simulink model "FailureAnalysis"  (R2018b)
settings: Solver=VariableStepAuto  StartTime=0.0  StopTime=10.0  RelTol=1e-3
libraries: powerlib x75, peGeneralControl x6, dspstat3 x6, sldrtlib x1
settings Model: Creator=hp  LastModifiedBy=hp

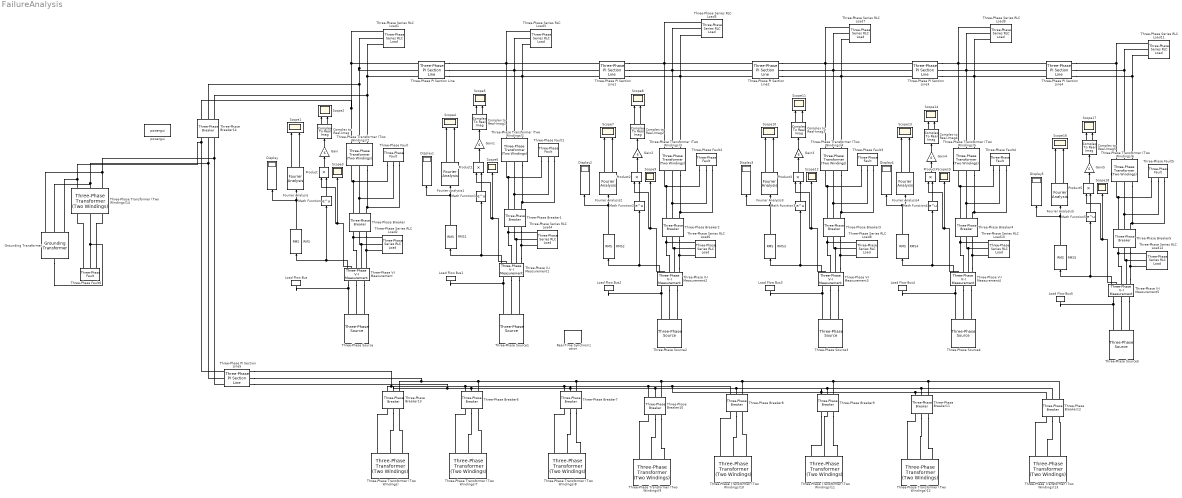
== system FailureAnalysis ==
  Complex to Real-Imag{,1..5} (6 alike) : ComplexToRealImag
  Display{,1..5} (6 alike) : Display
  Fourier Analysis{,1..5} (6 alike) : peGeneralControl/Fourier Analysis  f=60  n=[1 2]  M0=1  Ph0=0  Ts=-1
  Gain{,1..5} (6 alike) : Gain  Gain=6
  "Grounding Transformer " : powerlib/Elements/Grounding Transformer   UNITS=pu  NominalPower="[100e6   60]"  NominalVoltage=25e3  ZeroSequenceImpedance_pu=[0.025 0.75]  MagnetizationBranch_pu=[500 500]  ZeroSequenceImpedance_SI=[0.052083 589.05]  MagnetizationBranch_SI=[1041.7 3.927e+005]  Measurements=None
      settings: SourceProductName=Simscape Power Systems  SourceProductBaseCode=PS
  Load Flow Bus : powerlib/Measurements/Load Flow Bus  LConnTagsString=a  Phases=single  Connectors=on one side  ID=BUS_1  Vbase=25e3  Vref=1  Vangle=0  VLF=1  VLFb=1  VLFc=1  angleLF=0  angleLFb=0  angleLFc=0
      settings: SourceProductName=Simscape Power Systems
  Load Flow Bus1 : powerlib/Measurements/Load Flow Bus  LConnTagsString=a  Phases=single  Connectors=on one side  ID=BUS_2  Vbase=25e3  Vref=1  Vangle=0  VLF=1  VLFb=1  VLFc=1  angleLF=0  angleLFb=0  angleLFc=0
      settings: SourceProductName=Simscape Power Systems
  Load Flow Bus2 : powerlib/Measurements/Load Flow Bus  LConnTagsString=a  Phases=single  Connectors=on one side  ID=BUS_3  Vbase=25e3  Vref=1  Vangle=0  VLF=1  VLFb=1  VLFc=1  angleLF=0  angleLFb=0  angleLFc=0
      settings: SourceProductName=Simscape Power Systems
  Load Flow Bus3 : powerlib/Measurements/Load Flow Bus  LConnTagsString=a  Phases=single  Connectors=on one side  ID=BUS_4  Vbase=25e3  Vref=1  Vangle=0  VLF=1  VLFb=1  VLFc=1  angleLF=0  angleLFb=0  angleLFc=0
      settings: SourceProductName=Simscape Power Systems
  Load Flow Bus4 : powerlib/Measurements/Load Flow Bus  LConnTagsString=a  Phases=single  Connectors=on one side  ID=BUS_5  Vbase=25e3  Vref=1  Vangle=0  VLF=1  VLFb=1  VLFc=1  angleLF=0  angleLFb=0  angleLFc=0
      settings: SourceProductName=Simscape Power Systems
  Load Flow Bus5 : powerlib/Measurements/Load Flow Bus  LConnTagsString=a  Phases=single  Connectors=on one side  ID=BUS_6  Vbase=25e3  Vref=1  Vangle=0  VLF=1  VLFb=1  VLFc=1  angleLF=0  angleLFb=0  angleLFc=0
      settings: SourceProductName=Simscape Power Systems
  Math Function{,1..5} (6 alike) : Math  SaturateOnIntegerOverflow=on
  Product{,1..5} (6 alike) : Product
  RMS{,1..5} (6 alike) : dspstat3/RMS  run=off  directionMode=Each column  dimension=1  InputProcessing=Columns as channels (frame based)  reset_popup=None
  Real-Time Synchronization : sldrtlib/Real-Time Synchronization  SampleTime=0.1  MaxMissedTicks=10  ShowMissedTicks=off  YieldWhenWaiting=off
  Scope{1..2,4..5,7..8,10..11,13..14,16..17} (12 alike) : Scope  NumInputPorts=2
  Scope{3,6,9,12,15,18} (6 alike) : Scope
  Three-Phase PI Section Line{,1..4} (5 alike) : powerlib/Elements/Three-Phase PI Section Line  LConnTagsString=a|b|c  RConnTagsString=A|B|C  Frequency=60  Resistances=[ 0.01273 0.3864]  Inductances="[ 0.9337e-3  4.1264e-3]"  Capacitances=[12.74e-9 7.751e-9]  Length=0.1
      settings: SourceProductName=Simscape Power Systems
  Three-Phase PI Section Line5 : powerlib/Elements/Three-Phase PI Section Line  LConnTagsString=a|b|c  RConnTagsString=A|B|C  Frequency=60  Resistances=[ 0.01273 0.3864]  Inductances="[ 0.9337e-3  4.1264e-3]"  Capacitances=[12.74e-9 7.751e-9]  Length=100
      settings: SourceProductName=Simscape Power Systems
  Three-Phase Series RLC Load{1..12} (12 alike) : powerlib/Elements/Three-Phase Series RLC Load  LConnTagsString=A|B|C  Configuration=Y (grounded)  NominalVoltage=(1000)*10.749  Vabc=[1e3 1e3 1e3]  Vabcp=[1e3 1e3 1e3]  NominalFrequency=60  UnbalancedPower=off  ActivePower=10e3  InductivePower=100  CapacitivePower=100  Pabc=[10e3 9e3 11e3]  QLabc=[100 90 110]  QCabc=[100 90 110]  Pabcp=[10e3 9e3 11e3]  QLabcp=[100 90 110]  QCabcp=[100 90 110]  Measurements=Branch voltages and currents  LoadType=constant PQ
  Three-Phase Transformer (Two Windings){,7..13} (8 alike) : powerlib/Elements/Three-Phase Transformer (Two Windings)  Winding1Connection=Yg  Winding2Connection=Yg  CoreType=Three single-phase transformers  SetSaturation=off  Hysteresis=off  DataFile='hysteresis'  SetInitialFlux=off  Measurements=None  UNITS=pu  NominalPower=[ 250e6 , 60 ]  Winding1=[ 735e3 , 0.002 , 0.08 ]  Winding2=[ 315e3 , 0.002 , 0.08 ]  Rm=500  Lm=500  L0=0.5  Saturation=[ 0,0 ; 0.0024,1.2 ; 1.0,1.52 ]  InitialFluxes=[ 0.8 , -0.8 , 0.7 ]  MoreParameters=off  BreakLoop=off  DataType=off  TransfoNumber=1
  Three-Phase Transformer (Two Windings){1..6} (6 alike) : powerlib/Elements/Three-Phase Transformer (Two Windings)  Winding1Connection=Yg  Winding2Connection=Yg  CoreType=Three single-phase transformers  SetSaturation=off  Hysteresis=off  DataFile='hysteresis'  SetInitialFlux=off  Measurements=All measurements (V I Fluxes)  UNITS=pu  NominalPower=[ 250e6 , 60 ]  Winding1=[ 735e3 , 0.002 , 0.08 ]  Winding2=[ 315e3 , 0.002 , 0.08 ]  Rm=500  Lm=500  L0=0.5  Saturation=[ 0,0 ; 0.0024,1.2 ; 1.0,1.52 ]  InitialFluxes=[ 0.8 , -0.8 , 0.7 ]  MoreParameters=off  BreakLoop=off  DataType=off  TransfoNumber=1
  Three-Phase Transformer (Two Windings)14 : powerlib/Elements/Three-Phase Transformer (Two Windings)  Winding1Connection=Yg  Winding2Connection=Yg  CoreType=Three single-phase transformers  SetSaturation=off  Hysteresis=off  DataFile='hysteresis'  SetInitialFlux=off  Measurements=None  UNITS=pu  NominalPower=[ 250e6 , 60 ]  Winding1=[ 17.5e3 , 0.002 , 0.08 ]  Winding2=[ 120 , 0.002 , 0.08 ]  Rm=500  Lm=500  L0=0.5  Saturation=[ 0,0 ; 0.0024,1.2 ; 1.0,1.52 ]  InitialFluxes=[ 0.8 , -0.8 , 0.7 ]  MoreParameters=off  BreakLoop=off  DataType=off  TransfoNumber=1
  Three-Phase V-I Measurement{,1..5} (6 alike) : powerlib/Measurements/Three-Phase V-I Measurement  VoltageMeasurement=phase-to-ground  SetLabelV=off  LabelV=Vabc  Vpu=on  VpuLL=off  CurrentMeasurement=yes  SetLabelI=off  LabelI=Iabc  Ipu=off  Pbase=100e6  Vbase=500e3  OutputType=Complex  PhasorSimulation=off  PSBequivalent=0
  Three-Phase Breaker{,1..14} (15 alike) : powerlib/Elements/Three-Phase Breaker  InitialState=closed  SwitchA=on  SwitchB=on  SwitchC=on  SwitchTimes="[1/60  5/60]"  External=off  BreakerResistance=0.01  SnubberResistance=1e6  SnubberCapacitance=inf  Measurements=None
  Three-Phase Fault{,1..5} (6 alike) : powerlib/Elements/Three-Phase Fault  InitialStates=0  FaultA=on  FaultB=on  FaultC=on  GroundFault=on  SwitchTimes="[1/60  5/60]"  External=off  SwitchStatus=NaN  FaultResistance=0.001  GroundResistance=0.01  SnubberResistance=1e6  SnubberCapacitance=inf  Measurements=Fault voltages
  Three-Phase Fault6 : powerlib/Elements/Three-Phase Fault  InitialStates=0  FaultA=on  FaultB=on  FaultC=on  GroundFault=on  SwitchTimes="[1/60  5/60]"  External=off  SwitchStatus=NaN  FaultResistance=0.001  GroundResistance=0.01  SnubberResistance=1e6  SnubberCapacitance=inf  Measurements=None
  Three-Phase Source{,1..5} (6 alike) : powerlib/Electrical Sources/Three-Phase Source  InternalConnection=Yg  VoltagePhases=off  Voltage=(25000)*0.999949  PhaseAngle=0.0058776  Voltage_phases=[25e3 25e3 25e3]/sqrt(3)  PhaseAngles_phases=[0 -120 +120]  Frequency=60  NonIdealSource=on  SpecifyImpedance=off  Resistance=0.8929  Inductance=16.58e-3  ShortCircuitLevel=100e6  BaseVoltage=25e3  XRratio=7  BusType=swing  Pref=7e6  Qref=0  Prefabc=[10e3, 10e3, 10e3]  Qrefabc=[0, 0, 0]  Qmin=-inf  Qmax=inf
  powergui : powerlib/powergui  Priority=1  SimulationMode=Continuous  SampleTime=50e-6  frequency=60  Iterations=50  frequencyindice=60  Pbase=7e6  ErrMax=0.0001  UnitsV=kV  UnitsW=MW  buscounter=0  FunctionMessages=off  echomessages=off  EnableUseOfTLC=off  CurrentSourceSwitches=off  DisableSnubberDevices=off  DisableRonSwitches=off  DisableVfSwitches=off  DisplayEquations=off  SolverType=Tustin/Backward Euler (TBE)  Interpol=off  ExternalGateDelay=off  methode=off  Ts=100  x0status=blocks  SPID=on  SwTol=0  HookPort=off  RestoreLinks=warning  ResistiveCurrentMeasurement=off  Frange=[0:2:500]  Ylog=off  Xlog=on  ShowGrid=off  save=off  variable=ZData  structure=0  ZoomFFT=off  StartTime=0.0  cycles=1  DisplayStyle=1  fundamental=60  FreqAxis=off  MaxFrequency=1000  frequencyindicesteady=60  RmsSteady=1  display=off
  wires:
  Math Function/1 -> Product/2
  Gain/1 -> Complex to Real-Imag/1
  Product/1 -> Gain/1
  RMS/1 -> Display/1, Fourier Analysis/1
  Fourier Analysis/2 -> Scope1/2
  Fourier Analysis/1 -> Scope1/1
  Complex to Real-Imag/1 -> Scope2/1
  Complex to Real-Imag/2 -> Scope2/2
  Three-Phase V-I Measurement/1 -> Math Function/1, RMS/1
  Three-Phase V-I Measurement/2 -> Product/1, Scope3/1
  Gain1/1 -> Complex to Real-Imag1/1
  Three-Phase V-I Measurement1/2 -> Product1/1, Scope6/1
  Three-Phase V-I Measurement1/1 -> Math Function1/1, RMS1/1
  Fourier Analysis1/1 -> Scope4/1
  Product1/1 -> Gain1/1
  Complex to Real-Imag1/1 -> Scope5/1
  Complex to Real-Imag1/2 -> Scope5/2
  Math Function1/1 -> Product1/2
  RMS1/1 -> Display1/1, Fourier Analysis1/1
  Fourier Analysis1/2 -> Scope4/2
  Gain2/1 -> Complex to Real-Imag2/1
  Three-Phase V-I Measurement2/2 -> Product2/1, Scope9/1
  Three-Phase V-I Measurement2/1 -> Math Function2/1, RMS2/1
  Fourier Analysis2/1 -> Scope7/1
  Product2/1 -> Gain2/1
  Complex to Real-Imag2/1 -> Scope8/1
  Complex to Real-Imag2/2 -> Scope8/2
  Math Function2/1 -> Product2/2
  RMS2/1 -> Display2/1, Fourier Analysis2/1
  Fourier Analysis2/2 -> Scope7/2
  Gain3/1 -> Complex to Real-Imag3/1
  Three-Phase V-I Measurement3/2 -> Product3/1, Scope12/1
  Three-Phase V-I Measurement3/1 -> Math Function3/1, RMS3/1
  Fourier Analysis3/1 -> Scope10/1
  Product3/1 -> Gain3/1
  Complex to Real-Imag3/1 -> Scope11/1
  Complex to Real-Imag3/2 -> Scope11/2
  Math Function3/1 -> Product3/2
  RMS3/1 -> Display3/1, Fourier Analysis3/1
  Fourier Analysis3/2 -> Scope10/2
  Math Function4/1 -> Product4/2
  Three-Phase V-I Measurement4/1 -> Math Function4/1, RMS4/1
  Fourier Analysis4/2 -> Scope13/2
  Product4/1 -> Gain4/1
  Complex to Real-Imag4/2 -> Scope14/2
  Three-Phase V-I Measurement4/2 -> Product4/1, Scope15/1
  RMS4/1 -> Display4/1, Fourier Analysis4/1
  Gain4/1 -> Complex to Real-Imag4/1
  Fourier Analysis4/1 -> Scope13/1
  Complex to Real-Imag4/1 -> Scope14/1
  Math Function5/1 -> Product5/2
  Three-Phase V-I Measurement5/1 -> Math Function5/1, RMS5/1
  Fourier Analysis5/2 -> Scope16/2
  Product5/1 -> Gain5/1
  Complex to Real-Imag5/2 -> Scope17/2
  Three-Phase V-I Measurement5/2 -> Product5/1, Scope18/1
  RMS5/1 -> Display5/1, Fourier Analysis5/1
  Gain5/1 -> Complex to Real-Imag5/1
  Fourier Analysis5/1 -> Scope16/1
  Complex to Real-Imag5/1 -> Scope17/1
  connections:
  Three-Phase V-I Measurement/LConn1 -- Three-Phase Source/RConn1 -- Load Flow Bus/LConn1
  Three-Phase V-I Measurement/LConn2 -- Three-Phase Source/RConn2
  Three-Phase V-I Measurement/LConn3 -- Three-Phase Source/RConn3
  Three-Phase Breaker/LConn3 -- Three-Phase Series RLC Load2/LConn3 -- Three-Phase V-I Measurement/RConn3
  Three-Phase V-I Measurement/RConn2 -- Three-Phase Breaker/LConn2 -- Three-Phase Series RLC Load2/LConn2
  Three-Phase Breaker/LConn1 -- Three-Phase V-I Measurement/RConn1 -- Three-Phase Series RLC Load2/LConn1
  Three-Phase Transformer (Two Windings)2/LConn3 -- Three-Phase Breaker/RConn3 -- Three-Phase Fault/LConn3
  Three-Phase Breaker/RConn2 -- Three-Phase Transformer (Two Windings)2/LConn2 -- Three-Phase Fault/LConn2
  Three-Phase Breaker/RConn1 -- Three-Phase Transformer (Two Windings)2/LConn1 -- Three-Phase Fault/LConn1
  Three-Phase Series RLC Load1/LConn2 -- Three-Phase PI Section Line/LConn2 -- Three-Phase Breaker14/RConn2 -- Three-Phase Transformer (Two Windings)2/RConn2
  Three-Phase Transformer (Two Windings)2/RConn1 -- Three-Phase Breaker14/RConn1 -- Three-Phase PI Section Line/LConn1 -- Three-Phase Series RLC Load1/LConn1
  Three-Phase Transformer (Two Windings)2/RConn3 -- Three-Phase Breaker14/RConn3 -- Three-Phase PI Section Line/LConn3 -- Three-Phase Series RLC Load1/LConn3
  Three-Phase Fault1/LConn3 -- Three-Phase Transformer (Two Windings)1/LConn3 -- Three-Phase Breaker1/RConn3
  Three-Phase Fault1/LConn2 -- Three-Phase Breaker1/RConn2 -- Three-Phase Transformer (Two Windings)1/LConn2
  Three-Phase V-I Measurement1/RConn3 -- Three-Phase Breaker1/LConn3 -- Three-Phase Series RLC Load4/LConn3
  Three-Phase Series RLC Load4/LConn2 -- Three-Phase Breaker1/LConn2 -- Three-Phase V-I Measurement1/RConn2
  Three-Phase Fault1/LConn1 -- Three-Phase Transformer (Two Windings)1/LConn1 -- Three-Phase Breaker1/RConn1
  Three-Phase Series RLC Load4/LConn1 -- Three-Phase V-I Measurement1/RConn1 -- Three-Phase Breaker1/LConn1
  Load Flow Bus1/LConn1 -- Three-Phase V-I Measurement1/LConn1 -- Three-Phase Source1/RConn1
  Three-Phase Transformer (Two Windings)1/RConn1 -- Three-Phase PI Section Line1/LConn1 -- Three-Phase Series RLC Load3/LConn1 -- Three-Phase PI Section Line/RConn1
  Three-Phase V-I Measurement1/LConn3 -- Three-Phase Source1/RConn3
  Three-Phase Transformer (Two Windings)1/RConn3 -- Three-Phase PI Section Line1/LConn3 -- Three-Phase PI Section Line/RConn3 -- Three-Phase Series RLC Load3/LConn3
  Three-Phase V-I Measurement1/LConn2 -- Three-Phase Source1/RConn2
  Three-Phase Series RLC Load3/LConn2 -- Three-Phase Transformer (Two Windings)1/RConn2 -- Three-Phase PI Section Line1/LConn2 -- Three-Phase PI Section Line/RConn2
  Three-Phase Fault2/LConn3 -- Three-Phase Transformer (Two Windings)3/LConn3 -- Three-Phase Breaker2/RConn3
  Three-Phase Fault2/LConn2 -- Three-Phase Breaker2/RConn2 -- Three-Phase Transformer (Two Windings)3/LConn2
  Three-Phase V-I Measurement2/RConn3 -- Three-Phase Breaker2/LConn3 -- Three-Phase Series RLC Load6/LConn3
  Three-Phase Series RLC Load6/LConn2 -- Three-Phase Breaker2/LConn2 -- Three-Phase V-I Measurement2/RConn2
  Three-Phase Fault2/LConn1 -- Three-Phase Transformer (Two Windings)3/LConn1 -- Three-Phase Breaker2/RConn1
  Three-Phase Series RLC Load6/LConn1 -- Three-Phase V-I Measurement2/RConn1 -- Three-Phase Breaker2/LConn1
  Load Flow Bus2/LConn1 -- Three-Phase V-I Measurement2/LConn1 -- Three-Phase Source2/RConn1
  Three-Phase Transformer (Two Windings)3/RConn1 -- Three-Phase Series RLC Load5/LConn1 -- Three-Phase PI Section Line2/LConn1 -- Three-Phase PI Section Line1/RConn1
  Three-Phase V-I Measurement2/LConn3 -- Three-Phase Source2/RConn3
  Three-Phase Transformer (Two Windings)3/RConn3 -- Three-Phase PI Section Line2/LConn3 -- Three-Phase PI Section Line1/RConn3 -- Three-Phase Series RLC Load5/LConn3
  Three-Phase V-I Measurement2/LConn2 -- Three-Phase Source2/RConn2
  Three-Phase Series RLC Load5/LConn2 -- Three-Phase Transformer (Two Windings)3/RConn2 -- Three-Phase PI Section Line2/LConn2 -- Three-Phase PI Section Line1/RConn2
  Three-Phase Fault3/LConn3 -- Three-Phase Transformer (Two Windings)4/LConn3 -- Three-Phase Breaker3/RConn3
  Three-Phase Fault3/LConn2 -- Three-Phase Breaker3/RConn2 -- Three-Phase Transformer (Two Windings)4/LConn2
  Three-Phase V-I Measurement3/RConn3 -- Three-Phase Breaker3/LConn3 -- Three-Phase Series RLC Load8/LConn3
  Three-Phase Series RLC Load8/LConn2 -- Three-Phase Breaker3/LConn2 -- Three-Phase V-I Measurement3/RConn2
  Three-Phase Fault3/LConn1 -- Three-Phase Transformer (Two Windings)4/LConn1 -- Three-Phase Breaker3/RConn1
  Three-Phase Series RLC Load8/LConn1 -- Three-Phase V-I Measurement3/RConn1 -- Three-Phase Breaker3/LConn1
  Load Flow Bus3/LConn1 -- Three-Phase V-I Measurement3/LConn1 -- Three-Phase Source3/RConn1
  Three-Phase Transformer (Two Windings)4/RConn1 -- Three-Phase Series RLC Load7/LConn1 -- Three-Phase PI Section Line3/LConn1 -- Three-Phase PI Section Line2/RConn1
  Three-Phase V-I Measurement3/LConn3 -- Three-Phase Source3/RConn3
  Three-Phase Transformer (Two Windings)4/RConn3 -- Three-Phase PI Section Line3/LConn3 -- Three-Phase PI Section Line2/RConn3 -- Three-Phase Series RLC Load7/LConn3
  Three-Phase V-I Measurement3/LConn2 -- Three-Phase Source3/RConn2
  Three-Phase Series RLC Load7/LConn2 -- Three-Phase Transformer (Two Windings)4/RConn2 -- Three-Phase PI Section Line3/LConn2 -- Three-Phase PI Section Line2/RConn2
  Three-Phase V-I Measurement4/RConn3 -- Three-Phase Breaker4/LConn3 -- Three-Phase Series RLC Load10/LConn3
  Three-Phase Series RLC Load10/LConn1 -- Three-Phase Breaker4/LConn1 -- Three-Phase V-I Measurement4/RConn1
  Load Flow Bus4/LConn1 -- Three-Phase V-I Measurement4/LConn1 -- Three-Phase Source4/RConn1
  Three-Phase Fault4/LConn3 -- Three-Phase Transformer (Two Windings)5/LConn3 -- Three-Phase Breaker4/RConn3
  Three-Phase Series RLC Load10/LConn2 -- Three-Phase V-I Measurement4/RConn2 -- Three-Phase Breaker4/LConn2
  Three-Phase Fault4/LConn2 -- Three-Phase Breaker4/RConn2 -- Three-Phase Transformer (Two Windings)5/LConn2
  Three-Phase Fault4/LConn1 -- Three-Phase Breaker4/RConn1 -- Three-Phase Transformer (Two Windings)5/LConn1
  Three-Phase V-I Measurement4/LConn3 -- Three-Phase Source4/RConn3
  Three-Phase Transformer (Two Windings)5/RConn3 -- Three-Phase PI Section Line4/LConn3 -- Three-Phase PI Section Line3/RConn3 -- Three-Phase Series RLC Load9/LConn3
  Three-Phase Series RLC Load9/LConn2 -- Three-Phase Transformer (Two Windings)5/RConn2 -- Three-Phase PI Section Line4/LConn2 -- Three-Phase PI Section Line3/RConn2
  Three-Phase Transformer (Two Windings)5/RConn1 -- Three-Phase PI Section Line4/LConn1 -- Three-Phase PI Section Line3/RConn1 -- Three-Phase Series RLC Load9/LConn1
  Three-Phase V-I Measurement4/LConn2 -- Three-Phase Source4/RConn2
  Three-Phase V-I Measurement5/RConn3 -- Three-Phase Breaker5/LConn3 -- Three-Phase Series RLC Load12/LConn3
  Three-Phase Series RLC Load12/LConn1 -- Three-Phase Breaker5/LConn1 -- Three-Phase V-I Measurement5/RConn1
  Load Flow Bus5/LConn1 -- Three-Phase V-I Measurement5/LConn1 -- Three-Phase Source5/RConn1
  Three-Phase Fault5/LConn3 -- Three-Phase Transformer (Two Windings)6/LConn3 -- Three-Phase Breaker5/RConn3
  Three-Phase Series RLC Load12/LConn2 -- Three-Phase V-I Measurement5/RConn2 -- Three-Phase Breaker5/LConn2
  Three-Phase Fault5/LConn2 -- Three-Phase Breaker5/RConn2 -- Three-Phase Transformer (Two Windings)6/LConn2
  Three-Phase Fault5/LConn1 -- Three-Phase Breaker5/RConn1 -- Three-Phase Transformer (Two Windings)6/LConn1
  Three-Phase V-I Measurement5/LConn3 -- Three-Phase Source5/RConn3
  Three-Phase Transformer (Two Windings)6/RConn3 -- Three-Phase PI Section Line4/RConn3 -- Three-Phase Series RLC Load11/LConn3
  Three-Phase Series RLC Load11/LConn2 -- Three-Phase PI Section Line4/RConn2 -- Three-Phase Transformer (Two Windings)6/RConn2
  Three-Phase Transformer (Two Windings)6/RConn1 -- Three-Phase Series RLC Load11/LConn1 -- Three-Phase PI Section Line4/RConn1
  Three-Phase V-I Measurement5/LConn2 -- Three-Phase Source5/RConn2
  Three-Phase Breaker6/RConn1 -- Three-Phase PI Section Line5/LConn1 -- Three-Phase Breaker13/RConn1 -- Three-Phase Breaker9/RConn1 -- Three-Phase Breaker12/RConn1 -- Three-Phase Breaker11/RConn1 -- Three-Phase Breaker8/RConn1 -- Three-Phase Breaker10/RConn1 -- Three-Phase Breaker7/RConn1
  Three-Phase Breaker7/RConn3 -- Three-Phase PI Section Line5/LConn2 -- Three-Phase Breaker13/RConn3 -- Three-Phase Breaker6/RConn3 -- Three-Phase Breaker12/RConn3 -- Three-Phase Breaker11/RConn3 -- Three-Phase Breaker9/RConn3 -- Three-Phase Breaker8/RConn3 -- Three-Phase Breaker10/RConn3
  Three-Phase Breaker8/RConn2 -- Three-Phase Breaker12/RConn2 -- Three-Phase Breaker11/RConn2 -- Three-Phase Breaker9/RConn2 -- Three-Phase PI Section Line5/LConn3 -- Three-Phase Breaker13/RConn2 -- Three-Phase Breaker6/RConn2 -- Three-Phase Breaker7/RConn2 -- Three-Phase Breaker10/RConn2
  Three-Phase Transformer (Two Windings)11/RConn2 -- Three-Phase Breaker9/LConn2
  Three-Phase Breaker9/LConn1 -- Three-Phase Transformer (Two Windings)11/RConn1
  Three-Phase Transformer (Two Windings)13/RConn3 -- Three-Phase Breaker12/LConn3
  Three-Phase Breaker11/LConn2 -- Three-Phase Transformer (Two Windings)12/RConn2
  Three-Phase Breaker9/LConn3 -- Three-Phase Transformer (Two Windings)11/RConn3
  Three-Phase Transformer (Two Windings)9/RConn1 -- Three-Phase Breaker10/LConn1
  Three-Phase Transformer (Two Windings)12/RConn1 -- Three-Phase Breaker11/LConn1
  Three-Phase Breaker8/LConn2 -- Three-Phase Transformer (Two Windings)10/RConn2
  Three-Phase Breaker10/LConn2 -- Three-Phase Transformer (Two Windings)9/RConn2
  Three-Phase Transformer (Two Windings)13/RConn1 -- Three-Phase Breaker12/LConn1
  Three-Phase Breaker7/LConn3 -- Three-Phase Transformer (Two Windings)8/RConn3
  Three-Phase Breaker10/LConn3 -- Three-Phase Transformer (Two Windings)9/RConn3
  Three-Phase Transformer (Two Windings)7/RConn3 -- Three-Phase Breaker6/LConn3
  Three-Phase Breaker13/LConn2 -- Three-Phase Transformer (Two Windings)/RConn2
  Three-Phase Breaker7/LConn2 -- Three-Phase Transformer (Two Windings)8/RConn2
  Three-Phase Transformer (Two Windings)8/RConn1 -- Three-Phase Breaker7/LConn1
  Three-Phase Breaker6/LConn2 -- Three-Phase Transformer (Two Windings)7/RConn2
  Three-Phase Transformer (Two Windings)10/RConn3 -- Three-Phase Breaker8/LConn3
  Three-Phase Breaker11/LConn3 -- Three-Phase Transformer (Two Windings)12/RConn3
  Three-Phase Transformer (Two Windings)/RConn1 -- Three-Phase Breaker13/LConn1
  Three-Phase Breaker12/LConn2 -- Three-Phase Transformer (Two Windings)13/RConn2
  Three-Phase Transformer (Two Windings)10/RConn1 -- Three-Phase Breaker8/LConn1
  Three-Phase Transformer (Two Windings)7/RConn1 -- Three-Phase Breaker6/LConn1
  Three-Phase Transformer (Two Windings)/RConn3 -- Three-Phase Breaker13/LConn3
  Three-Phase Transformer (Two Windings)14/RConn1 -- Three-Phase Breaker14/LConn1 -- Three-Phase PI Section Line5/RConn1 -- "Grounding Transformer "/LConn1
  Three-Phase Transformer (Two Windings)14/LConn2 -- Three-Phase Fault6/LConn2 -- "Grounding Transformer "/RConn1
  Three-Phase PI Section Line5/RConn3 -- "Grounding Transformer "/LConn3 -- Three-Phase Transformer (Two Windings)14/RConn3 -- Three-Phase Breaker14/LConn3
  Three-Phase PI Section Line5/RConn2 -- "Grounding Transformer "/LConn2 -- Three-Phase Transformer (Two Windings)14/RConn2 -- Three-Phase Breaker14/LConn2
  Three-Phase Fault6/LConn1 -- Three-Phase Transformer (Two Windings)14/LConn1
  Three-Phase Fault6/LConn3 -- Three-Phase Transformer (Two Windings)14/LConn3
